simulink model "Exp_8_batch_3_simulation"  (R2020a)
settings: Solver=ode45  StartTime=0.0  StopTime=2  RelTol=1e-3  EnableMultiTasking=on
InitFcn:
  | % Motor Parameters
  | Ra=2;                % Armature resistance in Ohms
  | La=5.2e-3;        %Armature Inductance in H
  | flux_e=0.1        %Back EMF and torque Conatant
  | J=1.5e-4;          %Constant of Inertia
  | Bm=1e-3;          %Frictional torque coefficient
  | 
  | % Torque Controller Parameters
  | 
  | Kpt=1.38;
  | Kit=5880;
  | sat_T=3;
  | 
  | % Speed Controller Parameter
  | 
  | Kpw=1.17;
  | Kiw=527;
  | sat_w=18;
Description:
  | This model simulates the position control of a DC motor.
  | 
  | Syed Abdul Rahman Kashif
  | UET, Lahore
settings Model: Creator=Abdul Rahman Kashif  LastModifiedBy=sundaram bhupathi
settings DataIOCC: LimitDataPoints=on  SaveFormat=Array  SignalLoggingSaveFormat=ModelDataLogs  ReturnWorkspaceOutputs=off
settings OptimizationCC: ExpressionDepthLimit=2147483647  LifeSpan=inf
settings DebuggingCC: UnderspecifiedInitializationDetection=Classic  MergeDetectMultiDrivingBlocksExec=none  SolverPrmCheckMsg=warning  FcnCallInpInsideContextMsg=warning  StateNameClashWarn=warning  SFUnexpectedBacktrackingDiag=warning  SFNoUnconditionalDefaultTransitionDiag=warning  SFExecutionAtInitializationDiag=none  ArithmeticOperatorsInVariantConditions=warning
settings HardwareCC: ProdBitPerPointer=32  ProdBitPerSizeT=32  ProdBitPerPtrDiffT=32  ProdLargestAtomicFloat=None  ProdIntDivRoundTo=Undefined  ProdEndianess=Unspecified  ProdWordSize=32  ProdHWDeviceType=32-bit Generic
settings ModelReferenceCC: PropagateSignalLabelsOutOfModel=off
settings SFSimCC: SimUseLocalCustomCode=off  CustomCodeUndefinedFunction=UseInterfaceOnly
settings RTWCC: RTWUseLocalCustomCode=off
settings CodeAppCC: StateflowObjectComments=on
settings GRTTargetCC: TargetLangStandard=C89/C90 (ANSI)  CombineOutputUpdateFcns=off  GRTInterface=on
settings ConfigComp: CovMetricSettings=dw  CovHtmlReporting=on  CovSaveCumulativeToWorkspaceVar=on  CovSaveSingleToWorkspaceVar=on  CovExternalEMLEnable=off

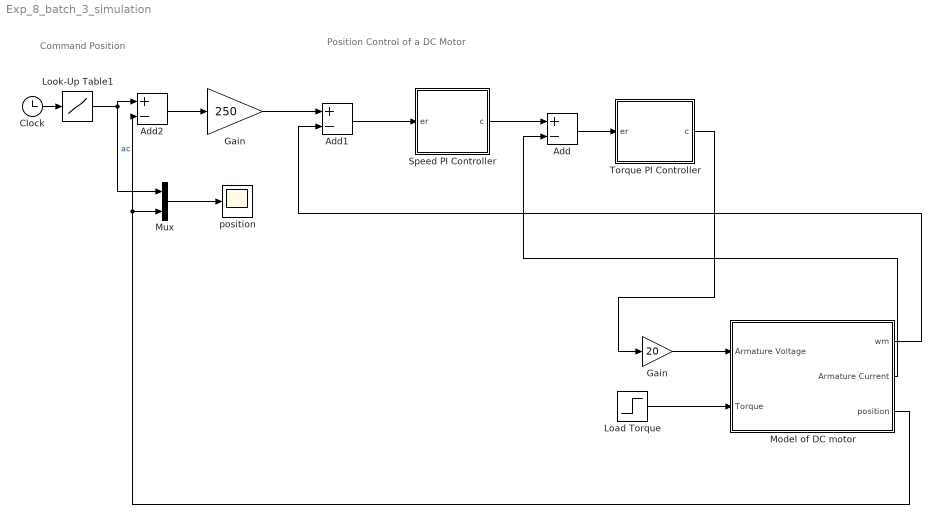
== system Exp_8_batch_3_simulation ==
  note: Position Control of a DC Motor
  note: Command Position
  Add : Sum  Inputs=+-
  Add1 : Sum  Inputs=+-
  Add2 : Sum  Inputs=+-
  Clock : Clock
  Gain : Gain  Gain=20
  "Gain " : Gain  Gain=250
  Load Torque : Step  Time=0.04  After=0.38  SampleTime=0
  Look-Up Table1 : Lookup  InputValues="[0  .05  .05 0.3 0.3 0.8 0.8 1.4 1.4 1.8]"  Table="[1 1 .5  .5 0.25 0.25 0.8 0.8 0.1 0.1]"  SaturateOnIntegerOverflow=on
  Model of DC motor : Subsystem
  Mux : Mux  Inputs=2
  Speed PI Controller : Subsystem
      mask Display: plot(0,0,100,100,[35,35,65],[70,30,30],[35,65],[45,60])
  Torque PI Controller : Subsystem
      mask Display: plot(0,0,100,100,[35,35,65],[70,30,30],[35,65],[45,60])
  position : Scope
  wires:
  Clock/1 -> Look-Up Table1/1
  Gain/1 -> Model of DC motor/1(Armature Voltage)
  Load Torque/1 -> Model of DC motor/2(Torque)
  Torque PI Controller/1(c) -> Gain/1
  Add/1 -> Torque PI Controller/1(er)
  Model of DC motor/2(Armature Current) -> Add/2
  Speed PI Controller/1(c) -> Add/1
  Add1/1 -> Speed PI Controller/1(er)
  Model of DC motor/1(wm) -> Add1/2
  "Gain "/1 -> Add1/1
  Add2/1 -> "Gain "/1
  Look-Up Table1/1 -> Add2/1, Mux/1  "ac"
  Model of DC motor/3(position) -> Add2/2, Mux/2
  Mux/1 -> position/1

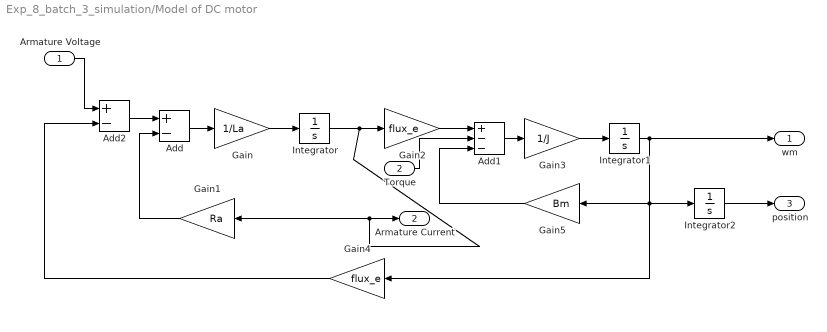
== system Exp_8_batch_3_simulation/Model of DC motor ==
  Armature Voltage : Inport
  Torque : Inport  Port=2
  Add : Sum  Inputs=+-
  Add1 : Sum  Inputs=+--
  Add2 : Sum  Inputs=+-
  Gain : Gain  Gain=1/La
  Gain1 : Gain  Gain=Ra
  Gain2 : Gain  Gain=flux_e
  Gain3 : Gain  Gain=1/J
  Gain4 : Gain  Gain=flux_e
  Gain5 : Gain  Gain=Bm
  Integrator : Integrator
  Integrator1 : Integrator
  Integrator2 : Integrator
  wm : Outport
  Armature Current : Outport  Port=2
  position : Outport  Port=3
  wires:
  Gain/1 -> Integrator/1
  Integrator/1 -> Gain2/1, Gain1/1, Armature Current/1
  Add/1 -> Gain/1
  Gain1/1 -> Add/2
  Gain2/1 -> Add1/1
  Add1/1 -> Gain3/1
  Gain3/1 -> Integrator1/1
  Add2/1 -> Add/1
  Gain4/1 -> Add2/2
  Integrator1/1 -> wm/1, Gain4/1, Integrator2/1, Gain5/1
  Torque/1 -> Add1/2
  Armature Voltage/1 -> Add2/1
  Gain5/1 -> Add1/3
  Integrator2/1 -> position/1

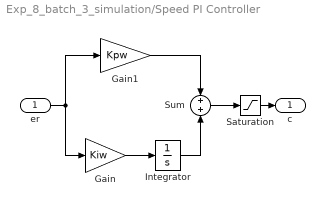
== system Exp_8_batch_3_simulation/Speed PI Controller ==
  er : Inport
  Gain : Gain  Gain=Kiw  SaturateOnIntegerOverflow=on  OutDataTypeStr=Inherit: Same as input  ParamDataTypeStr=Inherit: Same as input
  Gain1 : Gain  Gain=Kpw  SaturateOnIntegerOverflow=on  OutDataTypeStr=Inherit: Same as input  ParamDataTypeStr=Inherit: Same as input
  Integrator : Integrator  LimitOutput=on  UpperSaturationLimit=sat_w  LowerSaturationLimit=-sat_w
  Saturation : Saturate  UpperLimit=sat_w  LowerLimit=-sat_w
  Sum : Sum  InputSameDT=on  SaturateOnIntegerOverflow=on  OutDataTypeStr=Inherit: Same as first input
  c : Outport  InitialOutput=0
  wires:
  Integrator/1 -> Sum/2
  Gain/1 -> Integrator/1
  Gain1/1 -> Sum/1
  er/1 -> Gain/1, Gain1/1
  Saturation/1 -> c/1
  Sum/1 -> Saturation/1

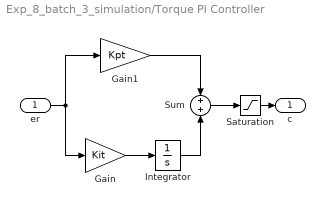
== system Exp_8_batch_3_simulation/Torque PI Controller ==
  er : Inport
  Gain : Gain  Gain=Kit  SaturateOnIntegerOverflow=on  OutDataTypeStr=Inherit: Same as input  ParamDataTypeStr=Inherit: Same as input
  Gain1 : Gain  Gain=Kpt  SaturateOnIntegerOverflow=on  OutDataTypeStr=Inherit: Same as input  ParamDataTypeStr=Inherit: Same as input
  Integrator : Integrator  LimitOutput=on  UpperSaturationLimit=sat_T  LowerSaturationLimit=-sat_T
  Saturation : Saturate  UpperLimit=sat_T  LowerLimit=-sat_T
  Sum : Sum  InputSameDT=on  SaturateOnIntegerOverflow=on  OutDataTypeStr=Inherit: Same as first input
  c : Outport  InitialOutput=0
  wires:
  Integrator/1 -> Sum/2
  Gain/1 -> Integrator/1
  Gain1/1 -> Sum/1
  er/1 -> Gain/1, Gain1/1
  Saturation/1 -> c/1
  Sum/1 -> Saturation/1
